simulink model "gm_combinedTxRx_AXIMM"  (R2017b)
settings: Solver=FixedStepDiscrete  StartTime=0.0  StopTime=10.0  RelTol=1e-3
InitFcn:
  | modelSettings
undefined symbols (not defined in the file or in its folder): coeff, filt, j, RadioSampleRate, VibertiTracebackLength, xPreambleSeq
libraries: hdlmdlgenlib x24, simulink x20, dsphdlfiltering x20, hdlsllib x10, dspsigops x5, commseqgen3 x4, commdigbbndpm3 x3, commcrc2 x2, commcnvcod2 x2, commsource2 x1, dspstat3 x1, dspmlti4 x1
(part 4 of 6)

== system gm_combinedTxRx_AXIMM/Combined TX and RX/Receiver HDL/Frame Recover/Barker Locate/Measure Phase Ambiguity/HDL Opt Complex FIR4 ==
  In1 : Inport  SampleTime=1e-06
  validIn : Inport  Port=2  SampleTime=1e-06
  Add : Sum  Inputs=+-  AccumDataTypeStr=fixdt(1,16,0)
  Complex to Real-Imag : ComplexToRealImag
  Discrete FIR Filter HDL Optimized : dsphdlfiltering/Discrete FIR Filter HDL Optimized  Numerator=real(Taps)  Sharing=off  SharingFactor=2  SimulateUsing=Code generation  roundingMode=Floor  overflowMode=off  CoefficientsDataTypeStr=Inherit: Same word length as input  CoefficientsMin=[]  CoefficientsMax=[]  OutputDataTypeStr=fixdt(1,16,0)  OutputMin=[]  OutputMax=[]  ValidInPort=on  ReadyPort=off
      settings: SourceProductName=DSP System Toolbox  SourceProductBaseCode=DS
  Discrete FIR Filter HDL Optimized1 : dsphdlfiltering/Discrete FIR Filter HDL Optimized  Numerator=imag(Taps)  Sharing=off  SharingFactor=2  SimulateUsing=Code generation  roundingMode=Floor  overflowMode=off  CoefficientsDataTypeStr=Inherit: Same word length as input  CoefficientsMin=[]  CoefficientsMax=[]  OutputDataTypeStr=fixdt(1,16,0)  OutputMin=[]  OutputMax=[]  ValidInPort=on  ReadyPort=off
      settings: SourceProductName=DSP System Toolbox  SourceProductBaseCode=DS
  Discrete FIR Filter HDL Optimized2 : dsphdlfiltering/Discrete FIR Filter HDL Optimized  Numerator=real(Taps)  Sharing=off  SharingFactor=2  SimulateUsing=Code generation  roundingMode=Floor  overflowMode=off  CoefficientsDataTypeStr=Inherit: Same word length as input  CoefficientsMin=[]  CoefficientsMax=[]  OutputDataTypeStr=fixdt(1,16,0)  OutputMin=[]  OutputMax=[]  ValidInPort=on  ReadyPort=off
      settings: SourceProductName=DSP System Toolbox  SourceProductBaseCode=DS
  Discrete FIR Filter HDL Optimized3 : dsphdlfiltering/Discrete FIR Filter HDL Optimized  Numerator=imag(Taps)  Sharing=off  SharingFactor=2  SimulateUsing=Code generation  roundingMode=Floor  overflowMode=off  CoefficientsDataTypeStr=Inherit: Same word length as input  CoefficientsMin=[]  CoefficientsMax=[]  OutputDataTypeStr=fixdt(1,16,0)  OutputMin=[]  OutputMax=[]  ValidInPort=on  ReadyPort=off
      settings: SourceProductName=DSP System Toolbox  SourceProductBaseCode=DS
  Logical Operator : Logic  Inputs=4  AllPortsSameDT=off  OutDataTypeStr=boolean
  Real-Imag to Complex : RealImagToComplex
  Subtract : Sum  OutDataTypeStr=int16
  Out1 : Outport
  validOut : Outport  Port=2
  wires:
  Add/1 -> Real-Imag to Complex/1
  Complex to Real-Imag/1 -> Discrete FIR Filter HDL Optimized/1, Discrete FIR Filter HDL Optimized3/1
  Complex to Real-Imag/2 -> Discrete FIR Filter HDL Optimized1/1, Discrete FIR Filter HDL Optimized2/1
  Discrete FIR Filter HDL Optimized/1 -> Add/1
  Discrete FIR Filter HDL Optimized/2 -> Logical Operator/1
  Discrete FIR Filter HDL Optimized1/1 -> Add/2
  Discrete FIR Filter HDL Optimized1/2 -> Logical Operator/2
  Discrete FIR Filter HDL Optimized2/1 -> Subtract/1
  Discrete FIR Filter HDL Optimized2/2 -> Logical Operator/3
  Discrete FIR Filter HDL Optimized3/1 -> Subtract/2
  Discrete FIR Filter HDL Optimized3/2 -> Logical Operator/4
  Logical Operator/1 -> validOut/1
  Real-Imag to Complex/1 -> Out1/1
  Subtract/1 -> Real-Imag to Complex/2
  In1/1 -> Complex to Real-Imag/1
  validIn/1 -> Discrete FIR Filter HDL Optimized/2, Discrete FIR Filter HDL Optimized1/2, Discrete FIR Filter HDL Optimized2/2, Discrete FIR Filter HDL Optimized3/2

== system gm_combinedTxRx_AXIMM/Combined TX and RX/Receiver HDL/Frame Recover/Barker Locate/Measure Phase Ambiguity/HDL Opt Complex FIR5 ==
  In1 : Inport  SampleTime=1e-06
  validIn : Inport  Port=2  SampleTime=1e-06
  Add : Sum  Inputs=+-  AccumDataTypeStr=fixdt(1,16,0)
  Complex to Real-Imag : ComplexToRealImag
  Discrete FIR Filter HDL Optimized : dsphdlfiltering/Discrete FIR Filter HDL Optimized  Numerator=real(Taps)  Sharing=off  SharingFactor=2  SimulateUsing=Code generation  roundingMode=Floor  overflowMode=off  CoefficientsDataTypeStr=Inherit: Same word length as input  CoefficientsMin=[]  CoefficientsMax=[]  OutputDataTypeStr=fixdt(1,16,0)  OutputMin=[]  OutputMax=[]  ValidInPort=on  ReadyPort=off
      settings: SourceProductName=DSP System Toolbox  SourceProductBaseCode=DS
  Discrete FIR Filter HDL Optimized1 : dsphdlfiltering/Discrete FIR Filter HDL Optimized  Numerator=imag(Taps)  Sharing=off  SharingFactor=2  SimulateUsing=Code generation  roundingMode=Floor  overflowMode=off  CoefficientsDataTypeStr=Inherit: Same word length as input  CoefficientsMin=[]  CoefficientsMax=[]  OutputDataTypeStr=fixdt(1,16,0)  OutputMin=[]  OutputMax=[]  ValidInPort=on  ReadyPort=off
      settings: SourceProductName=DSP System Toolbox  SourceProductBaseCode=DS
  Discrete FIR Filter HDL Optimized2 : dsphdlfiltering/Discrete FIR Filter HDL Optimized  Numerator=real(Taps)  Sharing=off  SharingFactor=2  SimulateUsing=Code generation  roundingMode=Floor  overflowMode=off  CoefficientsDataTypeStr=Inherit: Same word length as input  CoefficientsMin=[]  CoefficientsMax=[]  OutputDataTypeStr=fixdt(1,16,0)  OutputMin=[]  OutputMax=[]  ValidInPort=on  ReadyPort=off
      settings: SourceProductName=DSP System Toolbox  SourceProductBaseCode=DS
  Discrete FIR Filter HDL Optimized3 : dsphdlfiltering/Discrete FIR Filter HDL Optimized  Numerator=imag(Taps)  Sharing=off  SharingFactor=2  SimulateUsing=Code generation  roundingMode=Floor  overflowMode=off  CoefficientsDataTypeStr=Inherit: Same word length as input  CoefficientsMin=[]  CoefficientsMax=[]  OutputDataTypeStr=fixdt(1,16,0)  OutputMin=[]  OutputMax=[]  ValidInPort=on  ReadyPort=off
      settings: SourceProductName=DSP System Toolbox  SourceProductBaseCode=DS
  Logical Operator : Logic  Inputs=4  AllPortsSameDT=off  OutDataTypeStr=boolean
  Real-Imag to Complex : RealImagToComplex
  Subtract : Sum  OutDataTypeStr=int16
  Out1 : Outport
  validOut : Outport  Port=2
  wires:
  Add/1 -> Real-Imag to Complex/1
  Complex to Real-Imag/1 -> Discrete FIR Filter HDL Optimized/1, Discrete FIR Filter HDL Optimized3/1
  Complex to Real-Imag/2 -> Discrete FIR Filter HDL Optimized1/1, Discrete FIR Filter HDL Optimized2/1
  Discrete FIR Filter HDL Optimized/1 -> Add/1
  Discrete FIR Filter HDL Optimized/2 -> Logical Operator/1
  Discrete FIR Filter HDL Optimized1/1 -> Add/2
  Discrete FIR Filter HDL Optimized1/2 -> Logical Operator/2
  Discrete FIR Filter HDL Optimized2/1 -> Subtract/1
  Discrete FIR Filter HDL Optimized2/2 -> Logical Operator/3
  Discrete FIR Filter HDL Optimized3/1 -> Subtract/2
  Discrete FIR Filter HDL Optimized3/2 -> Logical Operator/4
  Logical Operator/1 -> validOut/1
  Real-Imag to Complex/1 -> Out1/1
  Subtract/1 -> Real-Imag to Complex/2
  In1/1 -> Complex to Real-Imag/1
  validIn/1 -> Discrete FIR Filter HDL Optimized/2, Discrete FIR Filter HDL Optimized1/2, Discrete FIR Filter HDL Optimized2/2, Discrete FIR Filter HDL Optimized3/2

== system gm_combinedTxRx_AXIMM/Combined TX and RX/Receiver HDL/Frame Recover/Barker Locate/Measure Phase Ambiguity/HDL Opt Complex FIR6 ==
  In1 : Inport  SampleTime=1e-06
  validIn : Inport  Port=2  SampleTime=1e-06
  Add : Sum  Inputs=+-  AccumDataTypeStr=fixdt(1,16,0)
  Complex to Real-Imag : ComplexToRealImag
  Discrete FIR Filter HDL Optimized : dsphdlfiltering/Discrete FIR Filter HDL Optimized  Numerator=real(Taps)  Sharing=off  SharingFactor=2  SimulateUsing=Code generation  roundingMode=Floor  overflowMode=off  CoefficientsDataTypeStr=Inherit: Same word length as input  CoefficientsMin=[]  CoefficientsMax=[]  OutputDataTypeStr=fixdt(1,16,0)  OutputMin=[]  OutputMax=[]  ValidInPort=on  ReadyPort=off
      settings: SourceProductName=DSP System Toolbox  SourceProductBaseCode=DS
  Discrete FIR Filter HDL Optimized1 : dsphdlfiltering/Discrete FIR Filter HDL Optimized  Numerator=imag(Taps)  Sharing=off  SharingFactor=2  SimulateUsing=Code generation  roundingMode=Floor  overflowMode=off  CoefficientsDataTypeStr=Inherit: Same word length as input  CoefficientsMin=[]  CoefficientsMax=[]  OutputDataTypeStr=fixdt(1,16,0)  OutputMin=[]  OutputMax=[]  ValidInPort=on  ReadyPort=off
      settings: SourceProductName=DSP System Toolbox  SourceProductBaseCode=DS
  Discrete FIR Filter HDL Optimized2 : dsphdlfiltering/Discrete FIR Filter HDL Optimized  Numerator=real(Taps)  Sharing=off  SharingFactor=2  SimulateUsing=Code generation  roundingMode=Floor  overflowMode=off  CoefficientsDataTypeStr=Inherit: Same word length as input  CoefficientsMin=[]  CoefficientsMax=[]  OutputDataTypeStr=fixdt(1,16,0)  OutputMin=[]  OutputMax=[]  ValidInPort=on  ReadyPort=off
      settings: SourceProductName=DSP System Toolbox  SourceProductBaseCode=DS
  Discrete FIR Filter HDL Optimized3 : dsphdlfiltering/Discrete FIR Filter HDL Optimized  Numerator=imag(Taps)  Sharing=off  SharingFactor=2  SimulateUsing=Code generation  roundingMode=Floor  overflowMode=off  CoefficientsDataTypeStr=Inherit: Same word length as input  CoefficientsMin=[]  CoefficientsMax=[]  OutputDataTypeStr=fixdt(1,16,0)  OutputMin=[]  OutputMax=[]  ValidInPort=on  ReadyPort=off
      settings: SourceProductName=DSP System Toolbox  SourceProductBaseCode=DS
  Logical Operator : Logic  Inputs=4  AllPortsSameDT=off  OutDataTypeStr=boolean
  Real-Imag to Complex : RealImagToComplex
  Subtract : Sum  OutDataTypeStr=int16
  Out1 : Outport
  validOut : Outport  Port=2
  wires:
  Add/1 -> Real-Imag to Complex/1
  Complex to Real-Imag/1 -> Discrete FIR Filter HDL Optimized/1, Discrete FIR Filter HDL Optimized3/1
  Complex to Real-Imag/2 -> Discrete FIR Filter HDL Optimized1/1, Discrete FIR Filter HDL Optimized2/1
  Discrete FIR Filter HDL Optimized/1 -> Add/1
  Discrete FIR Filter HDL Optimized/2 -> Logical Operator/1
  Discrete FIR Filter HDL Optimized1/1 -> Add/2
  Discrete FIR Filter HDL Optimized1/2 -> Logical Operator/2
  Discrete FIR Filter HDL Optimized2/1 -> Subtract/1
  Discrete FIR Filter HDL Optimized2/2 -> Logical Operator/3
  Discrete FIR Filter HDL Optimized3/1 -> Subtract/2
  Discrete FIR Filter HDL Optimized3/2 -> Logical Operator/4
  Logical Operator/1 -> validOut/1
  Real-Imag to Complex/1 -> Out1/1
  Subtract/1 -> Real-Imag to Complex/2
  In1/1 -> Complex to Real-Imag/1
  validIn/1 -> Discrete FIR Filter HDL Optimized/2, Discrete FIR Filter HDL Optimized1/2, Discrete FIR Filter HDL Optimized2/2, Discrete FIR Filter HDL Optimized3/2

== system gm_combinedTxRx_AXIMM/Combined TX and RX/Receiver HDL/Frame Recover/Barker Locate/Measure Phase Ambiguity/HDL Opt Complex FIR7 ==
  In1 : Inport  SampleTime=1e-06
  validIn : Inport  Port=2  SampleTime=1e-06
  Add : Sum  Inputs=+-  AccumDataTypeStr=fixdt(1,16,0)
  Complex to Real-Imag : ComplexToRealImag
  Discrete FIR Filter HDL Optimized : dsphdlfiltering/Discrete FIR Filter HDL Optimized  Numerator=real(Taps)  Sharing=off  SharingFactor=2  SimulateUsing=Code generation  roundingMode=Floor  overflowMode=off  CoefficientsDataTypeStr=Inherit: Same word length as input  CoefficientsMin=[]  CoefficientsMax=[]  OutputDataTypeStr=fixdt(1,16,0)  OutputMin=[]  OutputMax=[]  ValidInPort=on  ReadyPort=off
      settings: SourceProductName=DSP System Toolbox  SourceProductBaseCode=DS
  Discrete FIR Filter HDL Optimized1 : dsphdlfiltering/Discrete FIR Filter HDL Optimized  Numerator=imag(Taps)  Sharing=off  SharingFactor=2  SimulateUsing=Code generation  roundingMode=Floor  overflowMode=off  CoefficientsDataTypeStr=Inherit: Same word length as input  CoefficientsMin=[]  CoefficientsMax=[]  OutputDataTypeStr=fixdt(1,16,0)  OutputMin=[]  OutputMax=[]  ValidInPort=on  ReadyPort=off
      settings: SourceProductName=DSP System Toolbox  SourceProductBaseCode=DS
  Discrete FIR Filter HDL Optimized2 : dsphdlfiltering/Discrete FIR Filter HDL Optimized  Numerator=real(Taps)  Sharing=off  SharingFactor=2  SimulateUsing=Code generation  roundingMode=Floor  overflowMode=off  CoefficientsDataTypeStr=Inherit: Same word length as input  CoefficientsMin=[]  CoefficientsMax=[]  OutputDataTypeStr=fixdt(1,16,0)  OutputMin=[]  OutputMax=[]  ValidInPort=on  ReadyPort=off
      settings: SourceProductName=DSP System Toolbox  SourceProductBaseCode=DS
  Discrete FIR Filter HDL Optimized3 : dsphdlfiltering/Discrete FIR Filter HDL Optimized  Numerator=imag(Taps)  Sharing=off  SharingFactor=2  SimulateUsing=Code generation  roundingMode=Floor  overflowMode=off  CoefficientsDataTypeStr=Inherit: Same word length as input  CoefficientsMin=[]  CoefficientsMax=[]  OutputDataTypeStr=fixdt(1,16,0)  OutputMin=[]  OutputMax=[]  ValidInPort=on  ReadyPort=off
      settings: SourceProductName=DSP System Toolbox  SourceProductBaseCode=DS
  Logical Operator : Logic  Inputs=4  AllPortsSameDT=off  OutDataTypeStr=boolean
  Real-Imag to Complex : RealImagToComplex
  Subtract : Sum  OutDataTypeStr=int16
  Out1 : Outport
  validOut : Outport  Port=2
  wires:
  Add/1 -> Real-Imag to Complex/1
  Complex to Real-Imag/1 -> Discrete FIR Filter HDL Optimized/1, Discrete FIR Filter HDL Optimized3/1
  Complex to Real-Imag/2 -> Discrete FIR Filter HDL Optimized1/1, Discrete FIR Filter HDL Optimized2/1
  Discrete FIR Filter HDL Optimized/1 -> Add/1
  Discrete FIR Filter HDL Optimized/2 -> Logical Operator/1
  Discrete FIR Filter HDL Optimized1/1 -> Add/2
  Discrete FIR Filter HDL Optimized1/2 -> Logical Operator/2
  Discrete FIR Filter HDL Optimized2/1 -> Subtract/1
  Discrete FIR Filter HDL Optimized2/2 -> Logical Operator/3
  Discrete FIR Filter HDL Optimized3/1 -> Subtract/2
  Discrete FIR Filter HDL Optimized3/2 -> Logical Operator/4
  Logical Operator/1 -> validOut/1
  Real-Imag to Complex/1 -> Out1/1
  Subtract/1 -> Real-Imag to Complex/2
  In1/1 -> Complex to Real-Imag/1
  validIn/1 -> Discrete FIR Filter HDL Optimized/2, Discrete FIR Filter HDL Optimized1/2, Discrete FIR Filter HDL Optimized2/2, Discrete FIR Filter HDL Optimized3/2

== system gm_combinedTxRx_AXIMM/Combined TX and RX/Receiver HDL/Frame Recover/Equalization and Demodulation/2 Bit Descrambler/MATLAB Function ==
  in0 : Inport  OutDataTypeStr=boolean  PortDimensions=[2]  SampleTime=1e-06
  in1 : Inport  Port=2  OutDataTypeStr=boolean  SampleTime=1e-06
  Enable_out4 : EnablePort  OutDataTypeStr=boolean
  MATLAB Function : Subsystem
  out0 : Outport  OutDataTypeStr=boolean  PortDimensions=[1 7]  InitialOutput=0
  out1 : Outport  Port=2  OutDataTypeStr=boolean  PortDimensions=[1 7]  InitialOutput=0
  wires:
  MATLAB Function/1(bufferA) -> out0/1
  MATLAB Function/2(bufferB) -> out1/1
  in0/1 -> MATLAB Function/1(bits)
  in1/1 -> MATLAB Function/2(reset)

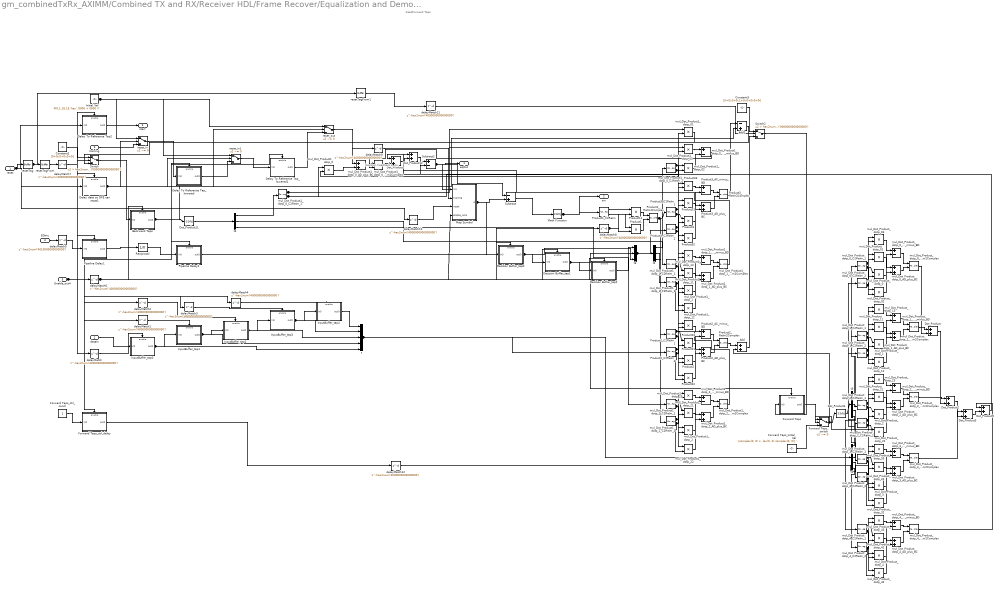
== system gm_combinedTxRx_AXIMM/Combined TX and RX/Receiver HDL/Frame Recover/Equalization and Demodulation/DFE/DFE ==
  note: Decision Feedback Taps
  note: FeedForward Taps
  reset : Inport  SampleTime=1e-06
  dataIn : Inport  Port=2  OutDataTypeStr=fixdt(1,16,14)  SampleTime=1e-06
  training : Inport  Port=3  OutDataTypeStr=fixdt(1,16,15)  SampleTime=1e-06
  EQmu : Inport  Port=4  SampleTime=1e-06
  Enable_out4 : Inport  Port=5  OutDataTypeStr=boolean  SampleTime=1e-06
  Add : Sum  AccumDataTypeStr=fixdt(1, 25, 22)  OutDataTypeStr=fixdt(1, 16, 14)  SampleTime=1e-06
  Add1 : Sum  Inputs=-+  AccumDataTypeStr=fixdt(1, 23, 21)  OutDataTypeStr=fixdt(1, 16, 19)  SampleTime=1e-06
  Backward Taps : Subsystem
      settings: MinAlgLoopOccurrences=on
  Constant2 : Constant  Value=[0+0i;0+0i;0+0i]  OutDataTypeStr=fixdt(1, 16, 4)  SampleTime=-1
  Constant3 : Constant  Value=[0+0i;0+0i;1+0i;0+0i;0+0i]  OutDataTypeStr=fixdt(1, 16, 4)  SampleTime=-1
  Decision Buffer_tap0 : Subsystem
      settings: MinAlgLoopOccurrences=on
  Decision Buffer_tap1 : Subsystem
      settings: MinAlgLoopOccurrences=on
  Decision Buffer_tap2 : Subsystem
      settings: MinAlgLoopOccurrences=on
  Delay To Reference Tap2 : Subsystem
      settings: MinAlgLoopOccurrences=on
  Delay To Reference Tap_lowered : Subsystem
      settings: MinAlgLoopOccurrences=on
  Delay To Reference Tap_lowered1 : Subsystem
      settings: MinAlgLoopOccurrences=on
  Delay data so DFE can reset1 : Subsystem
      settings: MinAlgLoopOccurrences=on
  Dot_Product{,2..3,5} (4 alike) : Sum  AccumDataTypeStr=fixdt(1, 16, 14)  OutDataTypeStr=fixdt(1, 16, 14)  SampleTime=1e-06  SaturateOnIntegerOverflow=on
  Dot_Product1 : Sum  AccumDataTypeStr=fixdt(1, 16, 18)  OutDataTypeStr=fixdt(1, 16, 18)  SampleTime=1e-06  SaturateOnIntegerOverflow=on
  Dot_Product11 : Math  Operator=conj  SaturateOnIntegerOverflow=on
  Dot_Product12 : Sum  AccumDataTypeStr=fixdt(1, 16, 18)  OutDataTypeStr=fixdt(1, 16, 18)  SampleTime=1e-06  SaturateOnIntegerOverflow=on
  Dot_Product4 : Math  Operator=conj  SaturateOnIntegerOverflow=on
  Forward Taps : Subsystem
      settings: MinAlgLoopOccurrences=on
  Forward Taps_Initial_Val : Constant  Value=[complex(0, 0) complex(0, 0) complex(1, 0) complex(0, 0) complex(0, 0)].'  OutDataTypeStr=fixdt(1, 16, 14)  SampleTime=-1
  Forward Taps_ctrl_const : Constant  OutDataTypeStr=boolean  SampleTime=1e-06
  Forward Taps_ctrl_delay : Subsystem
      settings: MinAlgLoopOccurrences=on
  Forward Taps_switch : Switch  Criteria=u2 ~= 0  Threshold=hex2num('0000000000000000')  OutDataTypeStr=fixdt(1, 16, 14)  SampleTime=1e-06
  Initial_Val : Constant  Value=fi(0,1,16,15,'hex','0000 + 0000 i')  OutDataTypeStr=fixdt(1, 16, 15)  SampleTime=-1
  InputBuffer_tap0 : Subsystem
      settings: MinAlgLoopOccurrences=on
  InputBuffer_tap1 : Subsystem
      settings: MinAlgLoopOccurrences=on
  InputBuffer_tap2 : Subsystem
      settings: MinAlgLoopOccurrences=on
  InputBuffer_tap3 : Subsystem
      settings: MinAlgLoopOccurrences=on
  InputBuffer_tap4 : Subsystem
      settings: MinAlgLoopOccurrences=on
  Map Symbol : Subsystem
  Math Function : Math  Operator=conj  RndMeth=Zero  SaturateOnIntegerOverflow=on
  Pipeline Delay1 : Subsystem
      settings: MinAlgLoopOccurrences=on
  Pipeline Delay2 : Subsystem
      settings: MinAlgLoopOccurrences=on
  Product{1..2,11,21..23} (6 alike) : Product  Inputs=**  OutDataTypeStr=fixdt(1, 16, 22)  SampleTime=1e-06
  Product1_C2ReIm : ComplexToRealImag  SampleTime=1e-06
  Product1_ReIm2Complex : RealImagToComplex  SampleTime=1e-06
  Product2_AC_minus_BD : Sum  Inputs=+-  OutDataTypeStr=fixdt(1, 16, 22)  SampleTime=1e-06
  Product2_AD_plus_BC : Sum  OutDataTypeStr=fixdt(1, 16, 22)  SampleTime=1e-06
  Product2_C2ReIm_1 : ComplexToRealImag  SampleTime=1e-06
  Product2_C2ReIm_2 : ComplexToRealImag  SampleTime=1e-06
  Product2_ReIm2Complex : RealImagToComplex  SampleTime=1e-06
  Product{3,31..33} (4 alike) : Product  Inputs=**  OutDataTypeStr=fixdt(1, 16, 21)  SampleTime=1e-06
  Product3_AC_minus_BD : Sum  Inputs=+-  OutDataTypeStr=fixdt(1, 16, 21)  SampleTime=1e-06
  Product3_AD_plus_BC : Sum  OutDataTypeStr=fixdt(1, 16, 21)  SampleTime=1e-06
  Product3_C2ReIm_1 : ComplexToRealImag  SampleTime=1e-06
  Product3_C2ReIm_2 : ComplexToRealImag  SampleTime=1e-06
  Product3_ReIm2Complex : RealImagToComplex  SampleTime=1e-06
  Reciprocal : Product  Inputs=/  OutDataTypeStr=fixdt(0, 16, 22)  SampleTime=1e-06  SaturateOnIntegerOverflow=on  RndMeth=Zero
  Subtract : Sum  Inputs=-+  AccumDataTypeStr=fixdt(1, 18, 15)  OutDataTypeStr=fixdt(1, 16, 15)  SampleTime=1e-06
  Subtract2 : Sum  Inputs=+-  AccumDataTypeStr=fixdt(1, 21, 18)  OutDataTypeStr=fixdt(1, 16, 14)  SampleTime=1e-06
  Switch : Switch  Criteria=u2 > Threshold  Threshold=hex2num('0000000000000000')  OutDataTypeStr=fixdt(1, 16, 15)  SampleTime=1e-06
  Switch2 : Switch  Criteria=u2 > Threshold  Threshold=hex2num('0000000000000000')  OutDataTypeStr=fixdt(1, 16, 14)  SampleTime=1e-06
  delayMatch{,1..4,6..12} (12 alike) : Delay  DelayLength=hex2num('4000000000000000')  InitialCondition=0  InputProcessing=Inherited
  delayMatch5 : Delay  DelayLength=hex2num('4010000000000000')  InitialCondition=0  InputProcessing=Inherited
  mul_Dot_Product1_dotp_{0..2,11..13,21..23} (9 alike) : Product  Inputs=**  OutDataTypeStr=fixdt(1, 16, 18)  SampleTime=1e-06  SaturateOnIntegerOverflow=on
  mul_Dot_Product1_dotp_01 : Product  Inputs=**  OutDataTypeStr=fixdt(1, 16, 18)  SampleTime=1e-06  SaturateOnIntegerOverflow=on
  mul_Dot_Product1_dotp_02 : Product  Inputs=**  OutDataTypeStr=fixdt(1, 16, 18)  SampleTime=1e-06  SaturateOnIntegerOverflow=on
  mul_Dot_Product1_dotp_03 : Product  Inputs=**  OutDataTypeStr=fixdt(1, 16, 18)  SampleTime=1e-06  SaturateOnIntegerOverflow=on
  mul_Dot_Product1_dotp_0_AC_minus_BD : Sum  Inputs=+-  OutDataTypeStr=fixdt(1, 16, 18)  SampleTime=1e-06  SaturateOnIntegerOverflow=on
  mul_Dot_Product1_dotp_0_AD_plus_BC : Sum  OutDataTypeStr=fixdt(1, 16, 18)  SampleTime=1e-06  SaturateOnIntegerOverflow=on
  mul_Dot_Product1_dotp_0_C2ReIm_1 : ComplexToRealImag  SampleTime=1e-06
  mul_Dot_Product1_dotp_0_C2ReIm_2 : ComplexToRealImag  SampleTime=1e-06
  mul_Dot_Product1_dotp_0_ReIm2Complex : RealImagToComplex  SampleTime=1e-06
  mul_Dot_Product1_dotp_1_AC_minus_BD : Sum  Inputs=+-  OutDataTypeStr=fixdt(1, 16, 18)  SampleTime=1e-06  SaturateOnIntegerOverflow=on
  mul_Dot_Product1_dotp_1_AD_plus_BC : Sum  OutDataTypeStr=fixdt(1, 16, 18)  SampleTime=1e-06  SaturateOnIntegerOverflow=on
  mul_Dot_Product1_dotp_1_C2ReIm_1 : ComplexToRealImag  SampleTime=1e-06
  mul_Dot_Product1_dotp_1_C2ReIm_2 : ComplexToRealImag  SampleTime=1e-06
  mul_Dot_Product1_dotp_1_ReIm2Complex : RealImagToComplex  SampleTime=1e-06
  mul_Dot_Product1_dotp_2_AC_minus_BD : Sum  Inputs=+-  OutDataTypeStr=fixdt(1, 16, 18)  SampleTime=1e-06  SaturateOnIntegerOverflow=on
  mul_Dot_Product1_dotp_2_AD_plus_BC : Sum  OutDataTypeStr=fixdt(1, 16, 18)  SampleTime=1e-06  SaturateOnIntegerOverflow=on
  mul_Dot_Product1_dotp_2_C2ReIm_1 : ComplexToRealImag  SampleTime=1e-06
  mul_Dot_Product1_dotp_2_C2ReIm_2 : ComplexToRealImag  SampleTime=1e-06
  mul_Dot_Product1_dotp_2_ReIm2Complex : RealImagToComplex  SampleTime=1e-06
  mul_Dot_Product_dotp_{0..4,11..13,21..23,31..33,41..43} (17 alike) : Product  Inputs=**  OutDataTypeStr=fixdt(1, 16, 14)  SampleTime=1e-06  SaturateOnIntegerOverflow=on
  mul_Dot_Product_dotp_01 : Product  Inputs=**  OutDataTypeStr=fixdt(1, 16, 14)  SampleTime=1e-06  SaturateOnIntegerOverflow=on
  mul_Dot_Product_dotp_02 : Product  Inputs=**  OutDataTypeStr=fixdt(1, 16, 14)  SampleTime=1e-06  SaturateOnIntegerOverflow=on
  mul_Dot_Product_dotp_03 : Product  Inputs=**  OutDataTypeStr=fixdt(1, 16, 14)  SampleTime=1e-06  SaturateOnIntegerOverflow=on
  mul_Dot_Product_dotp_0_AC_minus_BD : Sum  Inputs=+-  OutDataTypeStr=fixdt(1, 16, 14)  SampleTime=1e-06  SaturateOnIntegerOverflow=on
  mul_Dot_Product_dotp_0_AD_plus_BC : Sum  OutDataTypeStr=fixdt(1, 16, 14)  SampleTime=1e-06  SaturateOnIntegerOverflow=on
  mul_Dot_Product_dotp_0_C2ReIm_1 : ComplexToRealImag  SampleTime=1e-06
  mul_Dot_Product_dotp_0_C2ReIm_2 : ComplexToRealImag  SampleTime=1e-06
  mul_Dot_Product_dotp_0_ReIm2Complex : RealImagToComplex  SampleTime=1e-06
  mul_Dot_Product_dotp_1_AC_minus_BD : Sum  Inputs=+-  OutDataTypeStr=fixdt(1, 16, 14)  SampleTime=1e-06  SaturateOnIntegerOverflow=on
  mul_Dot_Product_dotp_1_AD_plus_BC : Sum  OutDataTypeStr=fixdt(1, 16, 14)  SampleTime=1e-06  SaturateOnIntegerOverflow=on
  mul_Dot_Product_dotp_1_C2ReIm_1 : ComplexToRealImag  SampleTime=1e-06
  mul_Dot_Product_dotp_1_C2ReIm_2 : ComplexToRealImag  SampleTime=1e-06
  mul_Dot_Product_dotp_1_ReIm2Complex : RealImagToComplex  SampleTime=1e-06
  mul_Dot_Product_dotp_2_AC_minus_BD : Sum  Inputs=+-  OutDataTypeStr=fixdt(1, 16, 14)  SampleTime=1e-06  SaturateOnIntegerOverflow=on
  mul_Dot_Product_dotp_2_AD_plus_BC : Sum  OutDataTypeStr=fixdt(1, 16, 14)  SampleTime=1e-06  SaturateOnIntegerOverflow=on
  mul_Dot_Product_dotp_2_C2ReIm_1 : ComplexToRealImag  SampleTime=1e-06
  mul_Dot_Product_dotp_2_C2ReIm_2 : ComplexToRealImag  SampleTime=1e-06
  mul_Dot_Product_dotp_2_ReIm2Complex : RealImagToComplex  SampleTime=1e-06
  mul_Dot_Product_dotp_3_AC_minus_BD : Sum  Inputs=+-  OutDataTypeStr=fixdt(1, 16, 14)  SampleTime=1e-06  SaturateOnIntegerOverflow=on
  mul_Dot_Product_dotp_3_AD_plus_BC : Sum  OutDataTypeStr=fixdt(1, 16, 14)  SampleTime=1e-06  SaturateOnIntegerOverflow=on
  mul_Dot_Product_dotp_3_C2ReIm_1 : ComplexToRealImag  SampleTime=1e-06
  mul_Dot_Product_dotp_3_C2ReIm_2 : ComplexToRealImag  SampleTime=1e-06
  mul_Dot_Product_dotp_3_ReIm2Complex : RealImagToComplex  SampleTime=1e-06
  mul_Dot_Product_dotp_4_AC_minus_BD : Sum  Inputs=+-  OutDataTypeStr=fixdt(1, 16, 14)  SampleTime=1e-06  SaturateOnIntegerOverflow=on
  mul_Dot_Product_dotp_4_AD_plus_BC : Sum  OutDataTypeStr=fixdt(1, 16, 14)  SampleTime=1e-06  SaturateOnIntegerOverflow=on
  mul_Dot_Product_dotp_4_C2ReIm_1 : ComplexToRealImag  SampleTime=1e-06
  mul_Dot_Product_dotp_4_C2ReIm_2 : ComplexToRealImag  SampleTime=1e-06
  mul_Dot_Product_dotp_4_ReIm2Complex : RealImagToComplex  SampleTime=1e-06
  resetTag : hdlmdlgenlib/Buffer
      settings: SourceProductName=HDL Coder  SourceProductBaseCode=HD
  resetTagFrom : hdlmdlgenlib/Buffer
      settings: SourceProductName=HDL Coder  SourceProductBaseCode=HD
  resetTagFrom1 : hdlmdlgenlib/Buffer
      settings: SourceProductName=HDL Coder  SourceProductBaseCode=HD
  reset_in : Switch  Criteria=u2 ~= 0  Threshold=hex2num('0000000000000000')  OutDataTypeStr=fixdt(1, 16, 15)  SampleTime=1e-06
  reset_in1 : Switch  Criteria=u2 ~= 0  Threshold=hex2num('0000000000000000')  OutDataTypeStr=fixdt(1, 16, 15)  SampleTime=1e-06
  reset_out : Switch  Criteria=u2 ~= 0  Threshold=hex2num('0000000000000000')  OutDataTypeStr=fixdt(1, 16, 15)  SampleTime=1e-06
  t : Mux  Inputs=5
  t1 : Demux  Outputs=5
  t2 : Demux  Outputs=3
  t3 : Mux  Inputs=3
  t4 : Demux  Outputs=3
  t5 : Demux  Outputs=5
  eqOut : Outport  InitialOutput=0
  err : Outport  Port=2  InitialOutput=0
  start : Outport  Port=3  InitialOutput=0
  wires:
  delayMatch10/1 -> Map Symbol/3(reset)
  delayMatch5/1 -> Pipeline Delay1/1(in0)
  Constant2/1 -> Switch/1
  Constant3/1 -> Switch2/1
  delayMatch9/1 -> Map Symbol/2(training)
  Delay To Reference Tap2/1(out0) -> start/1
  Delay data so DFE can reset1/1(out0) -> reset_out/2, reset_in1/2, reset_in/2
  t/1 -> Product2_C2ReIm_2/1, t1/1
  Pipeline Delay1/1(out0) -> Reciprocal/1
  delayMatch8/1 -> Product1/2, Product11/2
  Reciprocal/1 -> Pipeline Delay2/1(in0)
  delayMatch7/1 -> Switch/2
  delayMatch11/1 -> Switch2/2
  resetTag/1 -> resetTagFrom1/1, resetTagFrom/1
  Forward Taps_Initial_Val/1 -> Forward Taps_switch/3
  Forward Taps_ctrl_const/1 -> Forward Taps_ctrl_delay/1(in0)
  delayMatch12/1 -> Forward Taps_switch/2
  Initial_Val/1 -> reset_out/1, reset_in1/1, reset_in/1
  Delay To Reference Tap_lowered/1(out0) -> reset_in1/3
  reset_in/1 -> Delay To Reference Tap_lowered/1(in0)
  Delay To Reference Tap_lowered1/1(out0) -> reset_out/3
  reset_in1/1 -> Delay To Reference Tap_lowered1/1(in0)
  InputBuffer_tap0/1(out0) -> InputBuffer_tap1/1(in0), t/5
  InputBuffer_tap1/1(out0) -> InputBuffer_tap2/1(in0), t/4
  InputBuffer_tap2/1(out0) -> InputBuffer_tap3/1(in0), t/3
  InputBuffer_tap3/1(out0) -> InputBuffer_tap4/1(in0), t/2
  InputBuffer_tap4/1(out0) -> t/1
  delayMatch/1 -> InputBuffer_tap0/Enable
  t1/1 -> mul_Dot_Product_dotp_0_C2ReIm_2/1
  t1/2 -> mul_Dot_Product_dotp_1_C2ReIm_2/1
  t1/3 -> mul_Dot_Product_dotp_2_C2ReIm_2/1
  t1/4 -> mul_Dot_Product_dotp_3_C2ReIm_2/1
  t1/5 -> mul_Dot_Product_dotp_4_C2ReIm_2/1
  mul_Dot_Product_dotp_0_C2ReIm_2/1 -> mul_Dot_Product_dotp_0/2, mul_Dot_Product_dotp_03/2
  mul_Dot_Product_dotp_0_C2ReIm_2/2 -> mul_Dot_Product_dotp_02/2, mul_Dot_Product_dotp_01/2
  mul_Dot_Product_dotp_1_C2ReIm_2/1 -> mul_Dot_Product_dotp_1/2, mul_Dot_Product_dotp_13/2
  mul_Dot_Product_dotp_1_C2ReIm_2/2 -> mul_Dot_Product_dotp_12/2, mul_Dot_Product_dotp_11/2
  mul_Dot_Product_dotp_2_C2ReIm_2/1 -> mul_Dot_Product_dotp_2/2, mul_Dot_Product_dotp_23/2
  mul_Dot_Product_dotp_2_C2ReIm_2/2 -> mul_Dot_Product_dotp_22/2, mul_Dot_Product_dotp_21/2
  mul_Dot_Product_dotp_3_C2ReIm_2/1 -> mul_Dot_Product_dotp_3/2, mul_Dot_Product_dotp_33/2
  mul_Dot_Product_dotp_3_C2ReIm_2/2 -> mul_Dot_Product_dotp_32/2, mul_Dot_Product_dotp_31/2
  mul_Dot_Product_dotp_4_C2ReIm_2/1 -> mul_Dot_Product_dotp_4/2, mul_Dot_Product_dotp_43/2
  mul_Dot_Product_dotp_4_C2ReIm_2/2 -> mul_Dot_Product_dotp_42/2, mul_Dot_Product_dotp_41/2
  Product2_C2ReIm_2/1 -> Product2/2, Product23/2
  Product2_C2ReIm_2/2 -> Product22/2, Product21/2
  reset/1 -> delayMatch10/1, Delay data so DFE can reset1/1(in0), Delay To Reference Tap2/1(in0), resetTag/1
  dataIn/1 -> InputBuffer_tap0/1(in0)
  training/1 -> reset_in/3
  EQmu/1 -> delayMatch5/1
  Enable_out4/1 -> delayMatch6/1, delayMatch4/1, delayMatch3/1, delayMatch2/1, delayMatch1/1, delayMatch/1, Delay To Reference Tap_lowered1/Enable, Delay To Reference Tap_lowered/Enable, Forward Taps_ctrl_delay/Enable, Pipeline Delay2/Enable, Pipeline Delay1/Enable, Delay data so DFE can reset1/Enable, Delay To Reference Tap2/Enable
  delayMatch1/1 -> InputBuffer_tap1/Enable
  delayMatch2/1 -> InputBuffer_tap2/Enable
  delayMatch3/1 -> InputBuffer_tap3/Enable
  delayMatch4/1 -> InputBuffer_tap4/Enable
  delayMatch6/1 -> Decision Buffer_tap2/Enable, Decision Buffer_tap1/Enable, Decision Buffer_tap0/Enable, Forward Taps/Enable, Backward Taps/Enable, Map Symbol/4(Enable_out4)
  resetTagFrom/1 -> delayMatch7/1
  Pipeline Delay2/1(out0) -> delayMatch8/1
  reset_out/1 -> delayMatch9/1
  resetTagFrom1/1 -> delayMatch11/1
  Forward Taps_ctrl_delay/1(out0) -> delayMatch12/1
  mul_Dot_Product1_dotp_0/1 -> mul_Dot_Product1_dotp_0_AD_plus_BC/2
  mul_Dot_Product1_dotp_01/1 -> mul_Dot_Product1_dotp_0_AD_plus_BC/1
  mul_Dot_Product1_dotp_0_AD_plus_BC/1 -> mul_Dot_Product1_dotp_0_ReIm2Complex/2
  mul_Dot_Product1_dotp_02/1 -> mul_Dot_Product1_dotp_0_AC_minus_BD/2
  mul_Dot_Product1_dotp_0_C2ReIm_2/1 -> mul_Dot_Product1_dotp_0/2, mul_Dot_Product1_dotp_03/2
  mul_Dot_Product1_dotp_0_C2ReIm_2/2 -> mul_Dot_Product1_dotp_02/2, mul_Dot_Product1_dotp_01/2
  mul_Dot_Product1_dotp_0_C2ReIm_1/1 -> mul_Dot_Product1_dotp_01/1, mul_Dot_Product1_dotp_03/1
  mul_Dot_Product1_dotp_0_C2ReIm_1/2 -> mul_Dot_Product1_dotp_0/1, mul_Dot_Product1_dotp_02/1
  mul_Dot_Product1_dotp_03/1 -> mul_Dot_Product1_dotp_0_AC_minus_BD/1
  mul_Dot_Product1_dotp_0_AC_minus_BD/1 -> mul_Dot_Product1_dotp_0_ReIm2Complex/1
  mul_Dot_Product1_dotp_0_ReIm2Complex/1 -> Dot_Product1/2
  mul_Dot_Product1_dotp_1/1 -> mul_Dot_Product1_dotp_1_AD_plus_BC/2
  mul_Dot_Product1_dotp_11/1 -> mul_Dot_Product1_dotp_1_AD_plus_BC/1
  mul_Dot_Product1_dotp_1_AD_plus_BC/1 -> mul_Dot_Product1_dotp_1_ReIm2Complex/2
  mul_Dot_Product1_dotp_12/1 -> mul_Dot_Product1_dotp_1_AC_minus_BD/2
  mul_Dot_Product1_dotp_1_C2ReIm_2/1 -> mul_Dot_Product1_dotp_1/2, mul_Dot_Product1_dotp_13/2
  mul_Dot_Product1_dotp_1_C2ReIm_2/2 -> mul_Dot_Product1_dotp_12/2, mul_Dot_Product1_dotp_11/2
  mul_Dot_Product1_dotp_1_C2ReIm_1/1 -> mul_Dot_Product1_dotp_11/1, mul_Dot_Product1_dotp_13/1
  mul_Dot_Product1_dotp_1_C2ReIm_1/2 -> mul_Dot_Product1_dotp_1/1, mul_Dot_Product1_dotp_12/1
  mul_Dot_Product1_dotp_13/1 -> mul_Dot_Product1_dotp_1_AC_minus_BD/1
  mul_Dot_Product1_dotp_1_AC_minus_BD/1 -> mul_Dot_Product1_dotp_1_ReIm2Complex/1
  mul_Dot_Product1_dotp_1_ReIm2Complex/1 -> Dot_Product1/1
  Dot_Product1/1 -> Dot_Product12/2
  mul_Dot_Product1_dotp_2/1 -> mul_Dot_Product1_dotp_2_AD_plus_BC/2
  mul_Dot_Product1_dotp_21/1 -> mul_Dot_Product1_dotp_2_AD_plus_BC/1
  mul_Dot_Product1_dotp_2_AD_plus_BC/1 -> mul_Dot_Product1_dotp_2_ReIm2Complex/2
  mul_Dot_Product1_dotp_22/1 -> mul_Dot_Product1_dotp_2_AC_minus_BD/2
  t2/1 -> mul_Dot_Product1_dotp_0_C2ReIm_2/1
  t2/2 -> mul_Dot_Product1_dotp_1_C2ReIm_2/1
  t2/3 -> mul_Dot_Product1_dotp_2_C2ReIm_2/1
  mul_Dot_Product1_dotp_2_C2ReIm_2/1 -> mul_Dot_Product1_dotp_2/2, mul_Dot_Product1_dotp_23/2
  mul_Dot_Product1_dotp_2_C2ReIm_2/2 -> mul_Dot_Product1_dotp_22/2, mul_Dot_Product1_dotp_21/2
  Product3/1 -> Product3_AD_plus_BC/2
  Product31/1 -> Product3_AD_plus_BC/1
  Product3_AD_plus_BC/1 -> Product3_ReIm2Complex/2
  Product32/1 -> Product3_AC_minus_BD/2
  Decision Buffer_tap0/1(out0) -> Decision Buffer_tap1/1(in0), t3/3
  Decision Buffer_tap1/1(out0) -> Decision Buffer_tap2/1(in0), t3/2
  Decision Buffer_tap2/1(out0) -> t3/1
  t3/1 -> Product3_C2ReIm_2/1, t2/1
  Product3_C2ReIm_2/1 -> Product3/2, Product33/2
  Product3_C2ReIm_2/2 -> Product32/2, Product31/2
  Product3_C2ReIm_1/1 -> Product31/1, Product33/1
  Product3_C2ReIm_1/2 -> Product3/1, Product32/1
  Product33/1 -> Product3_AC_minus_BD/1
  Product3_AC_minus_BD/1 -> Product3_ReIm2Complex/1
  Product3_ReIm2Complex/1 -> Add1/1
  Add1/1 -> Switch/3
  Switch/1 -> Backward Taps/1(in0)
  Backward Taps/1(out0) -> Dot_Product11/1, Add1/2
  Dot_Product11/1 -> t4/1
  t4/1 -> mul_Dot_Product1_dotp_0_C2ReIm_1/1
  t4/2 -> mul_Dot_Product1_dotp_1_C2ReIm_1/1
  t4/3 -> mul_Dot_Product1_dotp_2_C2ReIm_1/1
  mul_Dot_Product1_dotp_2_C2ReIm_1/1 -> mul_Dot_Product1_dotp_21/1, mul_Dot_Product1_dotp_23/1
  mul_Dot_Product1_dotp_2_C2ReIm_1/2 -> mul_Dot_Product1_dotp_2/1, mul_Dot_Product1_dotp_22/1
  mul_Dot_Product1_dotp_23/1 -> mul_Dot_Product1_dotp_2_AC_minus_BD/1
  mul_Dot_Product1_dotp_2_AC_minus_BD/1 -> mul_Dot_Product1_dotp_2_ReIm2Complex/1
  mul_Dot_Product1_dotp_2_ReIm2Complex/1 -> Dot_Product12/1
  Dot_Product12/1 -> Subtract2/2
  mul_Dot_Product_dotp_0/1 -> mul_Dot_Product_dotp_0_AD_plus_BC/2
  mul_Dot_Product_dotp_01/1 -> mul_Dot_Product_dotp_0_AD_plus_BC/1
  mul_Dot_Product_dotp_0_AD_plus_BC/1 -> mul_Dot_Product_dotp_0_ReIm2Complex/2
  mul_Dot_Product_dotp_02/1 -> mul_Dot_Product_dotp_0_AC_minus_BD/2
  mul_Dot_Product_dotp_0_C2ReIm_1/1 -> mul_Dot_Product_dotp_01/1, mul_Dot_Product_dotp_03/1
  mul_Dot_Product_dotp_0_C2ReIm_1/2 -> mul_Dot_Product_dotp_0/1, mul_Dot_Product_dotp_02/1
  mul_Dot_Product_dotp_03/1 -> mul_Dot_Product_dotp_0_AC_minus_BD/1
  mul_Dot_Product_dotp_0_AC_minus_BD/1 -> mul_Dot_Product_dotp_0_ReIm2Complex/1
  mul_Dot_Product_dotp_0_ReIm2Complex/1 -> Dot_Product/2
  mul_Dot_Product_dotp_1/1 -> mul_Dot_Product_dotp_1_AD_plus_BC/2
  mul_Dot_Product_dotp_11/1 -> mul_Dot_Product_dotp_1_AD_plus_BC/1
  mul_Dot_Product_dotp_1_AD_plus_BC/1 -> mul_Dot_Product_dotp_1_ReIm2Complex/2
  mul_Dot_Product_dotp_12/1 -> mul_Dot_Product_dotp_1_AC_minus_BD/2
  mul_Dot_Product_dotp_1_C2ReIm_1/1 -> mul_Dot_Product_dotp_11/1, mul_Dot_Product_dotp_13/1
  mul_Dot_Product_dotp_1_C2ReIm_1/2 -> mul_Dot_Product_dotp_1/1, mul_Dot_Product_dotp_12/1
  mul_Dot_Product_dotp_13/1 -> mul_Dot_Product_dotp_1_AC_minus_BD/1
  mul_Dot_Product_dotp_1_AC_minus_BD/1 -> mul_Dot_Product_dotp_1_ReIm2Complex/1
  mul_Dot_Product_dotp_1_ReIm2Complex/1 -> Dot_Product/1
  Dot_Product/1 -> Dot_Product2/2
  mul_Dot_Product_dotp_2/1 -> mul_Dot_Product_dotp_2_AD_plus_BC/2
  mul_Dot_Product_dotp_21/1 -> mul_Dot_Product_dotp_2_AD_plus_BC/1
  mul_Dot_Product_dotp_2_AD_plus_BC/1 -> mul_Dot_Product_dotp_2_ReIm2Complex/2
  mul_Dot_Product_dotp_22/1 -> mul_Dot_Product_dotp_2_AC_minus_BD/2
  mul_Dot_Product_dotp_2_C2ReIm_1/1 -> mul_Dot_Product_dotp_21/1, mul_Dot_Product_dotp_23/1
  mul_Dot_Product_dotp_2_C2ReIm_1/2 -> mul_Dot_Product_dotp_2/1, mul_Dot_Product_dotp_22/1
  mul_Dot_Product_dotp_23/1 -> mul_Dot_Product_dotp_2_AC_minus_BD/1
  mul_Dot_Product_dotp_2_AC_minus_BD/1 -> mul_Dot_Product_dotp_2_ReIm2Complex/1
  mul_Dot_Product_dotp_2_ReIm2Complex/1 -> Dot_Product2/1
  Dot_Product2/1 -> Dot_Product3/2
  mul_Dot_Product_dotp_3/1 -> mul_Dot_Product_dotp_3_AD_plus_BC/2
  mul_Dot_Product_dotp_31/1 -> mul_Dot_Product_dotp_3_AD_plus_BC/1
  mul_Dot_Product_dotp_3_AD_plus_BC/1 -> mul_Dot_Product_dotp_3_ReIm2Complex/2
  mul_Dot_Product_dotp_32/1 -> mul_Dot_Product_dotp_3_AC_minus_BD/2
  mul_Dot_Product_dotp_3_C2ReIm_1/1 -> mul_Dot_Product_dotp_31/1, mul_Dot_Product_dotp_33/1
  mul_Dot_Product_dotp_3_C2ReIm_1/2 -> mul_Dot_Product_dotp_3/1, mul_Dot_Product_dotp_32/1
  mul_Dot_Product_dotp_33/1 -> mul_Dot_Product_dotp_3_AC_minus_BD/1
  mul_Dot_Product_dotp_3_AC_minus_BD/1 -> mul_Dot_Product_dotp_3_ReIm2Complex/1
  mul_Dot_Product_dotp_3_ReIm2Complex/1 -> Dot_Product3/1
  Dot_Product3/1 -> Dot_Product5/2
  mul_Dot_Product_dotp_4/1 -> mul_Dot_Product_dotp_4_AD_plus_BC/2
  mul_Dot_Product_dotp_41/1 -> mul_Dot_Product_dotp_4_AD_plus_BC/1
  mul_Dot_Product_dotp_4_AD_plus_BC/1 -> mul_Dot_Product_dotp_4_ReIm2Complex/2
  mul_Dot_Product_dotp_42/1 -> mul_Dot_Product_dotp_4_AC_minus_BD/2
  Product2/1 -> Product2_AD_plus_BC/2
  Product21/1 -> Product2_AD_plus_BC/1
  Product2_AD_plus_BC/1 -> Product2_ReIm2Complex/2
  Product22/1 -> Product2_AC_minus_BD/2
  Product1/1 -> Product1_ReIm2Complex/2
  Map Symbol/1(d) -> Subtract/2, Decision Buffer_tap0/1(in0)
  Subtract/1 -> Math Function/1
  Product1_C2ReIm/1 -> Product11/1
  Product1_C2ReIm/2 -> Product1/1
  Product11/1 -> Product1_ReIm2Complex/1
  Product1_ReIm2Complex/1 -> Product3_C2ReIm_1/1, Product2_C2ReIm_1/1
  Product2_C2ReIm_1/1 -> Product21/1, Product23/1
  Product2_C2ReIm_1/2 -> Product2/1, Product22/1
  Product23/1 -> Product2_AC_minus_BD/1
  Product2_AC_minus_BD/1 -> Product2_ReIm2Complex/1
  Product2_ReIm2Complex/1 -> Add/1
  Add/1 -> Switch2/3
  Switch2/1 -> Forward Taps/1(in0)
  Forward Taps/1(out0) -> Forward Taps_switch/1
  Forward Taps_switch/1 -> Dot_Product4/1, Add/2
  Dot_Product4/1 -> t5/1
  t5/1 -> mul_Dot_Product_dotp_0_C2ReIm_1/1
  t5/2 -> mul_Dot_Product_dotp_1_C2ReIm_1/1
  t5/3 -> mul_Dot_Product_dotp_2_C2ReIm_1/1
  t5/4 -> mul_Dot_Product_dotp_3_C2ReIm_1/1
  t5/5 -> mul_Dot_Product_dotp_4_C2ReIm_1/1
  mul_Dot_Product_dotp_4_C2ReIm_1/1 -> mul_Dot_Product_dotp_41/1, mul_Dot_Product_dotp_43/1
  mul_Dot_Product_dotp_4_C2ReIm_1/2 -> mul_Dot_Product_dotp_4/1, mul_Dot_Product_dotp_42/1
  mul_Dot_Product_dotp_43/1 -> mul_Dot_Product_dotp_4_AC_minus_BD/1
  mul_Dot_Product_dotp_4_AC_minus_BD/1 -> mul_Dot_Product_dotp_4_ReIm2Complex/1
  mul_Dot_Product_dotp_4_ReIm2Complex/1 -> Dot_Product5/1
  Dot_Product5/1 -> Subtract2/1
  Math Function/1 -> Product1_C2ReIm/1, err/1
  Subtract2/1 -> Subtract/1, Map Symbol/1(In1), eqOut/1

== system gm_combinedTxRx_AXIMM/Combined TX and RX/Receiver HDL/Frame Recover/Equalization and Demodulation/DFE/Delay data so DFE can reset ==
  in0 : Inport  OutDataTypeStr=fixdt(1, 16, 14)  SampleTime=1e-06
      settings: SignalType=complex
  Enable_out4 : EnablePort  OutDataTypeStr=boolean
  Delay data so DFE can reset : Delay  DelayLength=hex2num('3ff0000000000000')  InitialCondition=0  InputProcessing=Inherited
  out0 : Outport  OutDataTypeStr=fixdt(1, 16, 14)  InitialOutput=0
      settings: SignalType=complex
  wires:
  Delay data so DFE can reset/1 -> out0/1
  in0/1 -> Delay data so DFE can reset/1

== system gm_combinedTxRx_AXIMM/Combined TX and RX/Receiver HDL/Frame Recover/Equalization and Demodulation/DFE/Delay ref so DFE can reset ==
  in0 : Inport  OutDataTypeStr=fixdt(1, 16, 15)  SampleTime=1e-06
      settings: SignalType=complex
  Enable_out4 : EnablePort  OutDataTypeStr=boolean
  Delay ref so DFE can reset : Delay  DelayLength=hex2num('3ff0000000000000')  InitialCondition=0  InputProcessing=Inherited
  out0 : Outport  OutDataTypeStr=fixdt(1, 16, 15)  InitialOutput=0
      settings: SignalType=complex
  wires:
  Delay ref so DFE can reset/1 -> out0/1
  in0/1 -> Delay ref so DFE can reset/1

== system gm_combinedTxRx_AXIMM/Combined TX and RX/Receiver HDL/Frame Recover/Equalization and Demodulation/DFE/PN Sequence Generator ==
  in0 : Inport  OutDataTypeStr=boolean  SampleTime=1e-06
  Enable_out4 : EnablePort  OutDataTypeStr=boolean
  PN Sequence Generator : commseqgen3/PN Sequence Generator  poly='z^5 + z^3 + z^1 + 1'  ini_sta=[1 1 1 0 0]  outBitMaskSource=Dialog parameter  shift=0  outVarSiz=off  maxOutSizeMode=Dialog parameter  maxOutSize=[10 1]  Ts=-1  sampPerFrame=1  reset=on  bitPackedOutputs=on  outDataType=Smallest unsigned integer  numPackedBits=2  bitPackDataSigned=off  bitPackedOutDType=Smallest integer
      settings: SourceProductName=Communications System Toolbox
  out0 : Outport  OutDataTypeStr=fixdt(0, 2, 0)  InitialOutput=0
  wires:
  PN Sequence Generator/1 -> out0/1
  in0/1 -> PN Sequence Generator/1

== system gm_combinedTxRx_AXIMM/Combined TX and RX/Receiver HDL/Frame Recover/Equalization and Demodulation/DFE/Packeted To Unpacked ==
  In1 : Inport  SampleTime=1e-06
  Extract Bits : simulink/Logic and Bit Operations/Extract Bits  bitsToExtract=Range of bits  numBits=8  bitIdxRange=[1]  outScalingMode=Treat bit field as an integer
      settings: SourceProductName=Simulink
  Extract Bits1 : simulink/Logic and Bit Operations/Extract Bits  bitsToExtract=Range of bits  numBits=8  bitIdxRange=[0]  outScalingMode=Treat bit field as an integer
      settings: SourceProductName=Simulink
  Vector Concatenate : Concatenate
  Out1 : Outport  InitialOutput=0
  wires:
  Extract Bits/1 -> Vector Concatenate/1
  Extract Bits1/1 -> Vector Concatenate/2
  Vector Concatenate/1 -> Out1/1
  In1/1 -> Extract Bits1/1, Extract Bits/1

== system gm_combinedTxRx_AXIMM/Combined TX and RX/Receiver HDL/Frame Recover/Equalization and Demodulation/DFE/QPSK Modulator Baseband ==
  in0 : Inport  OutDataTypeStr=fixdt(0, 1, 0)  PortDimensions=[2]  SampleTime=1e-06
  Enable_out4 : EnablePort  OutDataTypeStr=boolean
  QPSK Modulator Baseband : commdigbbndpm3/QPSK Modulator Baseband  InType=Bit  Enc=Binary  Ph=pi/4  outDtype=Fixed-point  outWordLen=16  outUDDataType=sfix(16)  outFracLenMode=User-defined  outFracLen=15  outDataTypeStr=fixdt(1,16,15)  outLastDataTypeStr=fixdt(1,16,15)
  out0 : Outport  OutDataTypeStr=fixdt(1, 16, 15)  InitialOutput=0
      settings: SignalType=complex
  wires:
  QPSK Modulator Baseband/1 -> out0/1
  in0/1 -> QPSK Modulator Baseband/1

== system gm_combinedTxRx_AXIMM/Combined TX and RX/Receiver HDL/Frame Recover/Equalization and Demodulation/Header Controller/Header Controller ==
  headerStart : Inport  SampleTime=1e-06
  data : Inport  Port=2  PortDimensions=2  SampleTime=1e-06
  RxTxFixedPointLibrary_c15_Header_Controller : MATLAB Function  TreatAsAtomicUnit=on
  enableDownstream : Outport  InitialOutput=0
  packetLenBitsOut : Outport  Port=2  InitialOutput=0
  resetViterbi : Outport  Port=3  InitialOutput=0
  crcStart : Outport  Port=4  InitialOutput=0
  status : Outport  Port=5  InitialOutput=0
  s1 : Outport  Port=6  InitialOutput=0
  s2 : Outport  Port=7  InitialOutput=0
  wires:
  headerStart/1 -> RxTxFixedPointLibrary_c15_Header_Controller/1(headerStart)
  data/1 -> RxTxFixedPointLibrary_c15_Header_Controller/2(data)
  RxTxFixedPointLibrary_c15_Header_Controller/1(enableDownstream) -> enableDownstream/1
  RxTxFixedPointLibrary_c15_Header_Controller/2(packetLenBitsOut) -> packetLenBitsOut/1
  RxTxFixedPointLibrary_c15_Header_Controller/3(resetViterbi) -> resetViterbi/1
  RxTxFixedPointLibrary_c15_Header_Controller/4(crcStart) -> crcStart/1
  RxTxFixedPointLibrary_c15_Header_Controller/5(status) -> status/1
  RxTxFixedPointLibrary_c15_Header_Controller/6(s1) -> s1/1
  RxTxFixedPointLibrary_c15_Header_Controller/7(s2) -> s2/1

== system gm_combinedTxRx_AXIMM/Combined TX and RX/Receiver HDL/Frame Recover/Frequency Recovery/Lock Detector/MATLAB Function ==
  u : Inport  SampleTime=1e-06
  RxTxFixedPointLibrary_c1_MATLAB_Function : MATLAB Function  TreatAsAtomicUnit=on
  y : Outport  InitialOutput=0
  wires:
  RxTxFixedPointLibrary_c1_MATLAB_Function/1(y) -> y/1
  u/1 -> RxTxFixedPointLibrary_c1_MATLAB_Function/1(u)

== system gm_combinedTxRx_AXIMM/Combined TX and RX/Receiver HDL/Frame Recover/Frequency Recovery/Lock Detector/Pipeline Delay ==
  in0 : Inport  OutDataTypeStr=fixdt(1, 16, 10)  SampleTime=1e-06
  Enable_out4 : EnablePort  OutDataTypeStr=boolean
  Pipeline Delay : Delay  DelayLength=hex2num('3ff0000000000000')  InitialCondition=0  InputProcessing=Inherited
  out0 : Outport  OutDataTypeStr=fixdt(1, 16, 10)  InitialOutput=0
  wires:
  Pipeline Delay/1 -> out0/1
  in0/1 -> Pipeline Delay/1

== system gm_combinedTxRx_AXIMM/Combined TX and RX/Receiver HDL/Frame Recover/Frequency Recovery/Lock Detector/Tapped Delay ==
  in0 : Inport  OutDataTypeStr=fixdt(0, 16, 10)  SampleTime=1e-06
  Enable_out4 : EnablePort  OutDataTypeStr=boolean
  Tapped Delay : simulink/Discrete/Tapped Delay  vinit=0  samptime=-1  NumDelays=hex2num('4059000000000000')  DelayOrder=Oldest  includeCurrent=off
  out0 : Outport  OutDataTypeStr=fixdt(0, 16, 10)  PortDimensions=[100]  InitialOutput=0
  wires:
  Tapped Delay/1 -> out0/1
  in0/1 -> Tapped Delay/1

== system gm_combinedTxRx_AXIMM/Combined TX and RX/Receiver HDL/Frame Recover/Frequency Recovery/Loop Filter Configurable/Delay ==
  in0 : Inport  OutDataTypeStr=fixdt(1, 16, 10)  SampleTime=1e-06
  Enable_out4 : EnablePort  OutDataTypeStr=boolean
  Delay : Delay  DelayLength=hex2num('3ff0000000000000')  InitialCondition=0  InputProcessing=Inherited
  out0 : Outport  OutDataTypeStr=fixdt(1, 16, 10)  InitialOutput=0
  wires:
  Delay/1 -> out0/1
  in0/1 -> Delay/1

== system gm_combinedTxRx_AXIMM/Combined TX and RX/Receiver HDL/Frame Recover/Frequency Recovery/Loop Filter Configurable/Delay3 ==
  in0 : Inport  OutDataTypeStr=fixdt(1, 16, 10)  SampleTime=1e-06
  Enable_out4 : EnablePort  OutDataTypeStr=boolean
  Delay3 : Delay  DelayLength=hex2num('3ff0000000000000')  InitialCondition=0  InputProcessing=Inherited
  out0 : Outport  OutDataTypeStr=fixdt(1, 16, 10)  InitialOutput=0
  wires:
  Delay3/1 -> out0/1
  in0/1 -> Delay3/1

== system gm_combinedTxRx_AXIMM/Combined TX and RX/Receiver HDL/Frame Recover/Frequency Recovery/Loop Filter Configurable/Delay4 ==
  in0 : Inport  OutDataTypeStr=fixdt(1, 16, 10)  SampleTime=1e-06
  Enable_out4 : EnablePort  OutDataTypeStr=boolean
  Delay4 : Delay  DelayLength=hex2num('3ff0000000000000')  InitialCondition=0  InputProcessing=Inherited
  out0 : Outport  OutDataTypeStr=fixdt(1, 16, 10)  InitialOutput=0
  wires:
  Delay4/1 -> out0/1
  in0/1 -> Delay4/1

== system gm_combinedTxRx_AXIMM/Combined TX and RX/Receiver HDL/Frame Recover/Gardner Timing Recovery/Gardner TED Blocks/Imag Error ==
  data : Inport  SampleTime=1e-06
  strobe sum : Inport  Port=2  SampleTime=1e-06
  Enable_out2 : Inport  Port=3  OutDataTypeStr=boolean  SampleTime=1e-06
  Delay : Subsystem
      settings: MinAlgLoopOccurrences=on
  Product1 : Product  Inputs=**  OutDataTypeStr=fixdt(1, 32, 20)  SampleTime=1e-06
  Sub : Sum  Inputs=+-  AccumDataTypeStr=fixdt(1, 16, 10)  OutDataTypeStr=fixdt(1, 16, 10)  SampleTime=1e-06
  TED Buffer Update1 : Subsystem
  Out1 : Outport  InitialOutput=0
  wires:
  data/1 -> Sub/2, Delay/1(in0)
  strobe sum/1 -> TED Buffer Update1/2(strobe sum)
  Delay/1(out0) -> TED Buffer Update1/1(new data)
  Product1/1 -> Out1/1
  Sub/1 -> Product1/2
  TED Buffer Update1/1(Middle Indx) -> Product1/1
  TED Buffer Update1/2(oldest) -> Sub/1
  Enable_out2/1 -> Delay/Enable, TED Buffer Update1/3(Enable_out2)

== system gm_combinedTxRx_AXIMM/Combined TX and RX/Receiver HDL/Frame Recover/Gardner Timing Recovery/Gardner TED Blocks/Real Error ==
  data : Inport  SampleTime=1e-06
  strobe sum : Inport  Port=2  SampleTime=1e-06
  Enable_out2 : Inport  Port=3  OutDataTypeStr=boolean  SampleTime=1e-06
  Delay : Subsystem
      settings: MinAlgLoopOccurrences=on
  Product1 : Product  Inputs=**  OutDataTypeStr=fixdt(1, 16, 12)  SampleTime=1e-06
  Sub : Sum  Inputs=+-  AccumDataTypeStr=fixdt(1, 16, 10)  OutDataTypeStr=fixdt(1, 16, 10)  SampleTime=1e-06
  TED Buffer Update1 : Subsystem
  Out1 : Outport  InitialOutput=0
  wires:
  data/1 -> Sub/2, Delay/1(in0)
  strobe sum/1 -> TED Buffer Update1/2(strobe sum)
  Delay/1(out0) -> TED Buffer Update1/1(new data)
  Product1/1 -> Out1/1
  Sub/1 -> Product1/2
  TED Buffer Update1/1(Middle Indx) -> Product1/1
  TED Buffer Update1/2(oldest) -> Sub/1
  Enable_out2/1 -> Delay/Enable, TED Buffer Update1/3(Enable_out2)

== system gm_combinedTxRx_AXIMM/Combined TX and RX/Receiver HDL/Frame Recover/Gardner Timing Recovery/Gardner TED Blocks/Strobe Buffer1_tap1 ==
  in0 : Inport  OutDataTypeStr=boolean  SampleTime=1e-06
  Enable_out2 : EnablePort  OutDataTypeStr=boolean
  Strobe Buffer1_tap1 : Delay  DelayLength=hex2num('3ff0000000000000')  InputProcessing=Inherited
  out0 : Outport  OutDataTypeStr=boolean  InitialOutput=0
  wires:
  Strobe Buffer1_tap1/1 -> out0/1
  in0/1 -> Strobe Buffer1_tap1/1

== system gm_combinedTxRx_AXIMM/Combined TX and RX/Receiver HDL/Frame Recover/Gardner Timing Recovery/Gardner TED Blocks/Strobe Buffer1_tap2 ==
  in0 : Inport  OutDataTypeStr=boolean  SampleTime=1e-06
  Enable_out2 : EnablePort  OutDataTypeStr=boolean
  Strobe Buffer1_tap2 : Delay  DelayLength=hex2num('3ff0000000000000')  InputProcessing=Inherited
  out0 : Outport  OutDataTypeStr=boolean  InitialOutput=0
  wires:
  Strobe Buffer1_tap2/1 -> out0/1
  in0/1 -> Strobe Buffer1_tap2/1

== system gm_combinedTxRx_AXIMM/Combined TX and RX/Receiver HDL/Frame Recover/Gardner Timing Recovery/Gardner TED Blocks/Strobe Buffer1_tap3 ==
  in0 : Inport  OutDataTypeStr=boolean  SampleTime=1e-06
  Enable_out2 : EnablePort  OutDataTypeStr=boolean
  Strobe Buffer1_tap3 : Delay  DelayLength=hex2num('3ff0000000000000')  InputProcessing=Inherited
  out0 : Outport  OutDataTypeStr=boolean  InitialOutput=0
  wires:
  Strobe Buffer1_tap3/1 -> out0/1
  in0/1 -> Strobe Buffer1_tap3/1
